simulink model "BPACPGLegDemo"  (R2025a)
settings: Solver=ode45  StartTime=0.0  StopTime=10  RelTol=1e-3
PreLoadFcn:
  | % --- knee model ---
  | I_knee = 0.06;      % kg*m^2 below-knee inertia
  | b_knee = 0.5;       % N*m*s/rad joint damping
  | K_knee = 0.5;       % N*m/rad return spring
  | th0    = 0.26;      % rad spring rest angle
  | ROM    = 1.5708;    % rad normalizing range
  | r_arm  = 0.035;     % m BPA moment arm
  | Tload  = 0.3;       % N*m constant flexion load
  | Fmax_ext = 500;     % N
  | Fmax_flex = 450;    % N
  | epsScale = 0.15;    % muscle strain span over ROM
  | % --- CPG (params tuned in tune_cpg2.m ODE prototype, 2026-09-10) ---
  | drive_ext  = 4.0;   % nA tonic drive to RG_ext (free V = -32 mV)
  | drive_flex = 3.6;   % nA tonic drive to RG_flex (asymmetry breaks the latch)
  | g_adp = 15;         % adaptive current at S_adp = 1 (nA)
  | tauAct = 50;        % ms muscle activation
libraries: SNS_Library x12
settings Model: Creator=Ben Bolen  LastModifiedBy=Ben Bolen

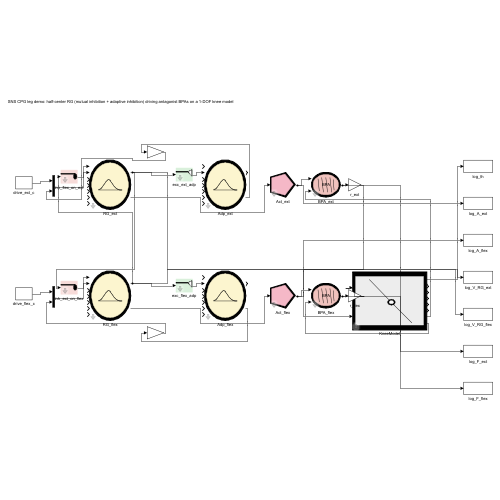
[thumbnail: Simulink's stored preview of the top-level diagram]
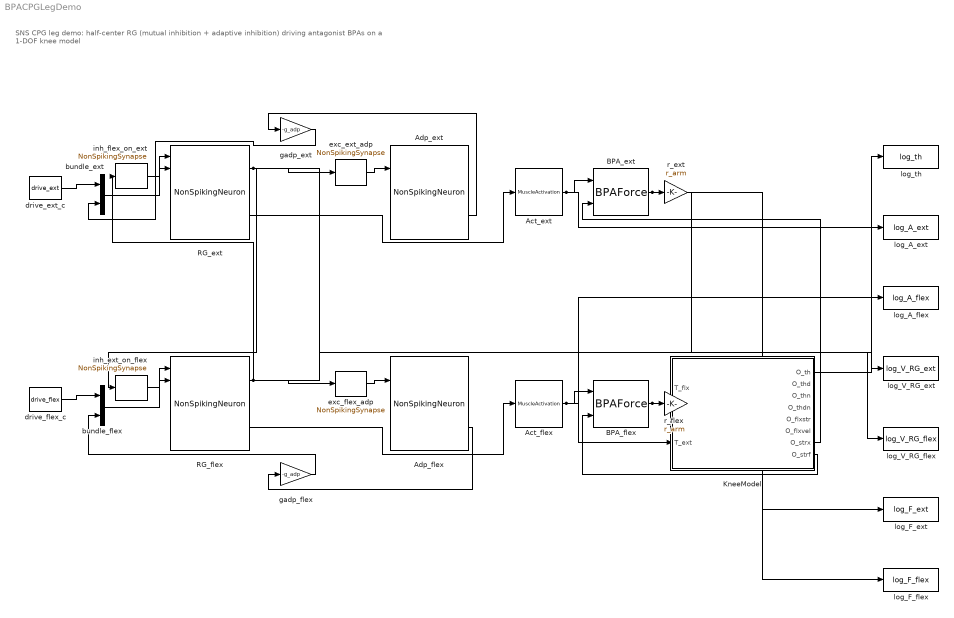
== system BPACPGLegDemo ==
  note: SNS CPG leg demo: half-center RG (mutual inhibition + adaptive inhibition) driving antagonist BPAs on a 1-DOF knee model
  Act_ext : SNS_Library/MuscleActivation  tauAct=50  A0=0
  Act_flex : SNS_Library/MuscleActivation  tauAct=50  A0=0
  Adp_ext : SNS_Library/NonSpikingNeuron  Vrest=-52  Gm=0.05  Cm=30  Thr=-45  Slope=1
  Adp_flex : SNS_Library/NonSpikingNeuron  Vrest=-52  Gm=0.05  Cm=30  Thr=-45  Slope=1
  BPA_ext : SNS_Library/BPAForce  Fmax=Fmax_ext  epsMax=0.25
  BPA_flex : SNS_Library/BPAForce  Fmax=Fmax_flex  epsMax=0.25
  KneeModel : Subsystem  mask(SNS Knee Model (1-DOF)){}
      mask help: Reduced-order 1-DOF knee: I*thdd = Tflex - Text + Tload - b*thd - K*(th-th0). theta = 0 deg full extension, +90 deg full flexion. Outputs theta, thd, and the normalized stretch/velocity/strain signals for the afferents.
      mask Display:
      | patch([-1 1 1 -1], [-1 -1 1 1], [0 0 0]);
      | patch([-0.92 0.92 0.92 -0.92], [-0.84 -0.84 0.84 0.84], [0.93 0.93 0.93]);
      | color('black');
      | plot([-0.55 0.05], [0.75 -0.05]);
      | plot([0.05 0.60], [-0.05 -0.75]);
      | t_ = linspace(0, 2*pi, 25);
      | patch(0.10*cos(t_) + 0.05, 0.10*sin(t_) - 0.05, [0 0 0]);
      | patch(0.055*cos(t_) + 0.05, 0.055*sin(t_) - 0.05, [1 1 1]);
  RG_ext : SNS_Library/NonSpikingNeuron  Vrest=-52  Gm=0.2  Cm=5  Thr=-45  Slope=1
  RG_flex : SNS_Library/NonSpikingNeuron  Vrest=-52  Gm=0.2  Cm=5  Thr=-45  Slope=1
  bundle_ext : Mux  Inputs=2
  bundle_flex : Mux  Inputs=2
  drive_ext_c : Constant  Value=drive_ext
  drive_flex_c : Constant  Value=drive_flex
  exc_ext_adp : SNS_Library/NonSpikingSynapse  gmax=0.12  Esyn=0  ThrPre=-45  SlopePre=0.5
  exc_flex_adp : SNS_Library/NonSpikingSynapse  gmax=0.12  Esyn=0  ThrPre=-45  SlopePre=0.5
  gadp_ext : Gain  Gain=-g_adp
  gadp_flex : Gain  Gain=-g_adp
  inh_ext_on_flex : SNS_Library/NonSpikingSynapse  gmax=0.8  Esyn=-72  ThrPre=-45  SlopePre=0.5
  inh_flex_on_ext : SNS_Library/NonSpikingSynapse  gmax=0.8  Esyn=-72  ThrPre=-45  SlopePre=0.5
  log_A_ext : ToWorkspace  VariableName=log_A_ext  SaveFormat=Timeseries  SampleTime=-1
  log_A_flex : ToWorkspace  VariableName=log_A_flex  SaveFormat=Timeseries  SampleTime=-1
  log_F_ext : ToWorkspace  VariableName=log_F_ext  SaveFormat=Timeseries  SampleTime=-1
  log_F_flex : ToWorkspace  VariableName=log_F_flex  SaveFormat=Timeseries  SampleTime=-1
  log_V_RG_ext : ToWorkspace  VariableName=log_V_RG_ext  SaveFormat=Timeseries  SampleTime=-1
  log_V_RG_flex : ToWorkspace  VariableName=log_V_RG_flex  SaveFormat=Timeseries  SampleTime=-1
  log_th : ToWorkspace  VariableName=log_th  SaveFormat=Timeseries  SampleTime=-1
  r_ext : Gain  Gain=r_arm
  r_flex : Gain  Gain=r_arm
  wires:
  drive_ext_c/1 -> bundle_ext/1
  gadp_ext/1 -> bundle_ext/2
  drive_flex_c/1 -> bundle_flex/1
  gadp_flex/1 -> bundle_flex/2
  bundle_ext/1 -> RG_ext/1
  bundle_flex/1 -> RG_flex/1
  RG_ext/1 -> inh_ext_on_flex/1, exc_ext_adp/1, log_V_RG_ext/1
  RG_flex/1 -> inh_flex_on_ext/1, exc_flex_adp/1, log_V_RG_flex/1
  inh_ext_on_flex/1 -> RG_flex/2
  inh_flex_on_ext/1 -> RG_ext/2
  exc_ext_adp/1 -> Adp_ext/2
  exc_flex_adp/1 -> Adp_flex/2
  Adp_ext/2 -> gadp_ext/1
  Adp_flex/2 -> gadp_flex/1
  RG_ext/2 -> Act_ext/1
  RG_flex/2 -> Act_flex/1
  Act_ext/1 -> BPA_ext/1, log_A_ext/1
  Act_flex/1 -> BPA_flex/1, log_A_flex/1
  BPA_flex/1 -> r_flex/1, log_F_flex/1
  BPA_ext/1 -> r_ext/1, log_F_ext/1
  r_flex/1 -> KneeModel/1(T_flx)
  r_ext/1 -> KneeModel/2(T_ext)
  KneeModel/7(O_strx) -> BPA_ext/2
  KneeModel/8(O_strf) -> BPA_flex/2
  KneeModel/1(O_th) -> log_th/1

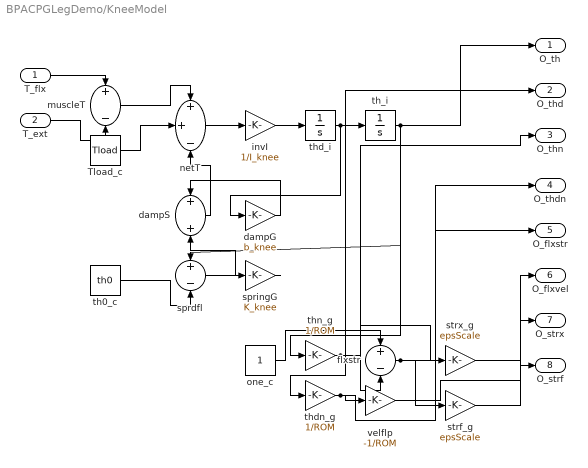
== system BPACPGLegDemo/KneeModel ==
  T_flx : Inport
  T_ext : Inport  Port=2
  Tload_c : Constant  Value=Tload
  dampG : Gain  Gain=b_knee
  dampS : Sum
  flxstr : Sum  Inputs=+-
  invI : Gain  Gain=1/I_knee
  muscleT : Sum  Inputs=+-
  netT : Sum  Inputs=++-
  one_c : Constant
  sprdfl : Sum  Inputs=+-
  springG : Gain  Gain=K_knee
  strf_g : Gain  Gain=epsScale
  strx_g : Gain  Gain=epsScale
  th0_c : Constant  Value=th0
  th_i : Integrator  InitialCondition=0.26
  thd_i : Integrator
  thdn_g : Gain  Gain=1/ROM
  thn_g : Gain  Gain=1/ROM
  velflp : Gain  Gain=-1/ROM
  O_th : Outport
  O_thd : Outport  Port=2
  O_thn : Outport  Port=3
  O_thdn : Outport  Port=4
  O_flxstr : Outport  Port=5
  O_flxvel : Outport  Port=6
  O_strx : Outport  Port=7
  O_strf : Outport  Port=8
  wires:
  strf_g/1 -> O_strf/1
  strx_g/1 -> O_strx/1
  velflp/1 -> O_flxvel/1
  flxstr/1 -> strf_g/1, O_flxstr/1
  one_c/1 -> flxstr/1
  thdn_g/1 -> velflp/1, O_thdn/1
  thn_g/1 -> strx_g/1, flxstr/2, O_thn/1
  springG/1 -> dampS/2
  dampG/1 -> dampS/1
  sprdfl/1 -> springG/1
  th0_c/1 -> sprdfl/2
  th_i/1 -> thn_g/1, O_th/1, sprdfl/1
  thd_i/1 -> thdn_g/1, O_thd/1, dampG/1, th_i/1
  invI/1 -> thd_i/1
  netT/1 -> invI/1
  dampS/1 -> netT/3
  Tload_c/1 -> netT/2
  muscleT/1 -> netT/1
  T_ext/1 -> muscleT/2
  T_flx/1 -> muscleT/1
